simulink model "TP1_Exercice_6_Cpt"  (R2023a)
settings: Solver=ode45  StartTime=0.0  StopTime=500  RelTol=1e-3  EnableMultiTasking=on
libraries: simulink_extras x4
settings Model: Creator=Steph  LastModifiedBy=e2300024
settings SolverCC: AlgebraicLoopSolver=TrustRegion
settings DataIOCC: LimitDataPoints=on  SaveFormat=Array  SignalLoggingSaveFormat=ModelDataLogs  ReturnWorkspaceOutputs=off
settings OptimizationCC: ExpressionDepthLimit=2147483647  LifeSpan=inf
settings DebuggingCC: UnderspecifiedInitializationDetection=Classic  MergeDetectMultiDrivingBlocksExec=none  SolverPrmCheckMsg=warning  FcnCallInpInsideContextMsg=warning  UnconnectedInputMsg=warning  UnconnectedOutputMsg=warning  UnconnectedLineMsg=warning  StateNameClashWarn=warning  SFUnexpectedBacktrackingDiag=warning  SFNoUnconditionalDefaultTransitionDiag=warning  SFExecutionAtInitializationDiag=none  ArithmeticOperatorsInVariantConditions=warning
settings HardwareCC: ProdBitPerPointer=32  ProdBitPerSizeT=32  ProdBitPerPtrDiffT=32  ProdLargestAtomicFloat=None  ProdIntDivRoundTo=Undefined  ProdEndianess=Unspecified  ProdWordSize=32  ProdHWDeviceType=32-bit Generic
settings ModelReferenceCC: PropagateSignalLabelsOutOfModel=off
settings SFSimCC: SimUseLocalCustomCode=off  CustomCodeUndefinedFunction=UseInterfaceOnly
settings RTWCC: RTWUseLocalCustomCode=off
settings CodeAppCC: StateflowObjectComments=on
settings GRTTargetCC: TargetLangStandard=C89/C90 (ANSI)
settings ConfigComp: CovMetricSettings=dw  CovSaveCumulativeToWorkspaceVar=on  CovSaveSingleToWorkspaceVar=on  CovExternalEMLEnable=off  CovSFcnEnable=off

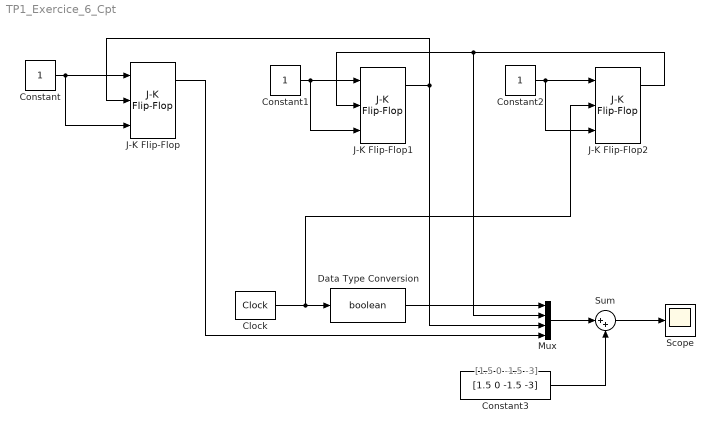
== system TP1_Exercice_6_Cpt ==
  note: [1.5 0 -1.5 -3]
  Clock : simulink_extras/Flip Flops/Clock  period=20
  Constant : Constant  OutDataTypeStr=boolean
  Constant1 : Constant  OutDataTypeStr=boolean
  Constant2 : Constant  OutDataTypeStr=boolean
  Constant3 : Constant  Value=[1.5 0 -1.5 -3]
  Data Type Conversion : DataTypeConversion  OutDataTypeStr=boolean  SaturateOnIntegerOverflow=off  RndMeth=Floor
  J-K Flip-Flop : simulink_extras/Flip Flops/J-K Flip-Flop  initial_condition=0
  J-K Flip-Flop1 : simulink_extras/Flip Flops/J-K Flip-Flop  initial_condition=0
  J-K Flip-Flop2 : simulink_extras/Flip Flops/J-K Flip-Flop  initial_condition=0
  Mux : Mux
  Scope : Scope
  Sum : Sum  Inputs=|++
  wires:
  Sum/1 -> Scope/1
  Constant3/1 -> Sum/2
  Mux/1 -> Sum/1
  Constant/1 -> J-K Flip-Flop/1, J-K Flip-Flop/3
  Constant1/1 -> J-K Flip-Flop1/1, J-K Flip-Flop1/3
  Constant2/1 -> J-K Flip-Flop2/1, J-K Flip-Flop2/3
  Clock/1 -> J-K Flip-Flop2/2, Data Type Conversion/1
  Data Type Conversion/1 -> Mux/1
  J-K Flip-Flop/1 -> Mux/4
  J-K Flip-Flop1/1 -> Mux/3, J-K Flip-Flop/2
  J-K Flip-Flop2/1 -> Mux/2, J-K Flip-Flop1/2
